simulink model "Bonus_1"  (R2024a)
settings: Solver=VariableStepAuto  StartTime=0.0  StopTime=10.0  RelTol=1e-3
libraries: HS_lib x124
settings Model: Creator=Anna  LastModifiedBy=Anna

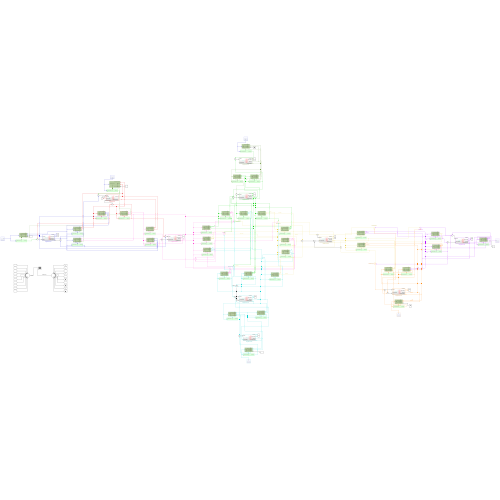
[thumbnail: Simulink's stored preview of the top-level diagram]
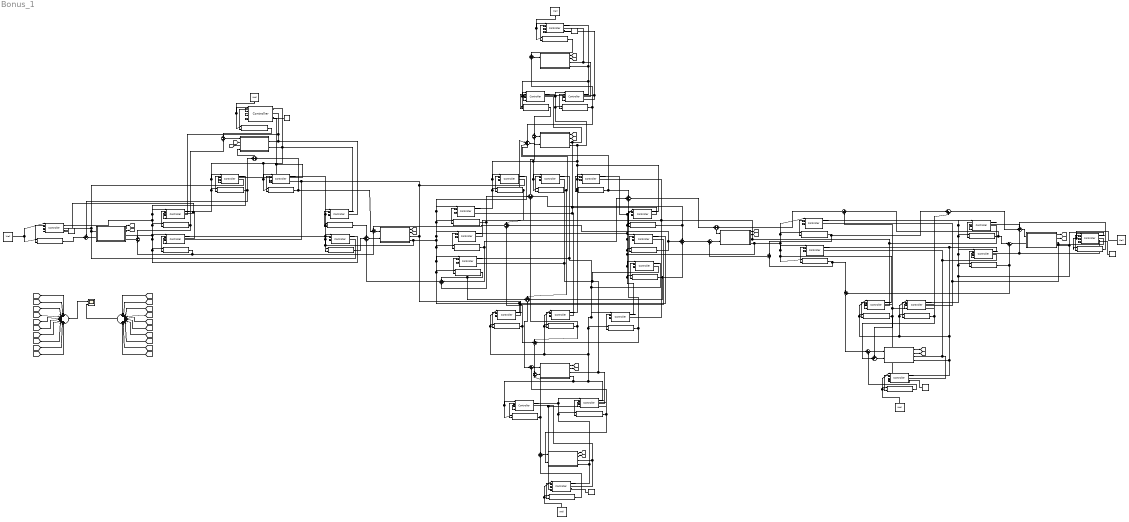
== system Bonus_1 ==
  Constant{,1..5} (6 alike) : Constant  Value=0
  Controller{1..34} (34 alike) : HS_lib/Controller  cn=0.4  cc=0.8  lb=0  ub=0
  From : From
  Goto2 : Goto
  INtakeYellow : Sum  Inputs=+++
  IntakeCyan : Sum  Inputs=+++
  IntakeGreen : Sum  Inputs=+++
  IntakeOrange : Sum  Inputs=|++
  IntakePink : Sum  Inputs=+++
  IntakeYellow2 : Sum  Inputs=|++
  Neighbourhood : Subsystem
      settings: PortSchema="{\"entries\":[{\"content\":{\"sides\":[{\"content\":{\"connectorIds\":[\"In1\",\"Out3\",\"Out4\",\"In2\"]},\"type\":\"ConnectorPlacement.EquallySpacedRectSide\",\"uuid\":\"a17f8f71-e2c0-4de1-9750-936e5df60ae2\"},{\"content\":{\"connectorIds\":[\"Out1\",\"Out2\"],\"side\":\"RIGHT\"},\"type\":\"ConnectorPlacement.EquallySpacedRectSide\",\"uuid\":\"d3f9e035-ab5e-46ba-a0b5-1d6a292e4fd8\"},{\"content\":{\"side\":\"TOP\"},\"type\":\"ConnectorPlacement.EquallySpacedRectSide\",\"uuid\":\"a414f663-cf97-4db1-b609-5e1d2eca4ce6\"}]},\"type\":\"ConnectorPlacement.EquallySpacedConnector\",\"uuid\":\"06d4f643-b53e-4a59-8698-2a41eae53feb\"}],\"packageUris\":[\"http://schema.mathworks.com/mf0/Connector/R2020b\"],\"version\":\"1.0\"}"
  Neighbourhood1 : Subsystem
      settings: PortSchema="{\"entries\":[{\"content\":{\"sides\":[{\"content\":{\"connectorIds\":[\"Out4\",\"In1\"]},\"type\":\"ConnectorPlacement.EquallySpacedRectSide\",\"uuid\":\"a17f8f71-e2c0-4de1-9750-936e5df60ae2\"},{\"content\":{\"connectorIds\":[\"Out1\",\"Out2\",\"Out3\",\"In2\"],\"side\":\"RIGHT\"},\"type\":\"ConnectorPlacement.EquallySpacedRectSide\",\"uuid\":\"d3f9e035-ab5e-46ba-a0b5-1d6a292e4fd8\"},{\"content\":{\"side\":\"TOP\"},\"type\":\"ConnectorPlacement.EquallySpacedRectSide\",\"uuid\":\"a414f663-cf97-4db1-b609-5e1d2eca4ce6\"}]},\"type\":\"ConnectorPlacement.EquallySpacedConnector\",\"uuid\":\"06d4f643-b53e-4a59-8698-2a41eae53feb\"}],\"packageUris\":[\"http://schema.mathworks.com/mf0/Connector/R2020b\"],\"version\":\"1.0\"}"
  Neighbourhood2 : Subsystem
  Neighbourhood3 : Subsystem
  Neighbourhood4 : Subsystem
  Neighbourhood5 : Subsystem
  Neighbourhood6 : Subsystem
  Neighbourhood7 : Subsystem
  Neighbourhood8 : Subsystem
  Neighbourhood9 : Subsystem
  Pump{1..34} (34 alike) : HS_lib/Pump  p=0
  Scope : Scope  NumInputPorts=2
  Sum{,1..2,7,9..10,12,14,17} (9 alike) : Sum
  Sum{11,13,16,19} (4 alike) : Sum  Inputs=|++
  Sum{4..6,15} (4 alike) : Sum  Inputs=+++
  Sum18 : Sum  Inputs=++|
  Sum20 : Sum  Inputs=++|
  Sum21 : Sum  Inputs=++++++++++
  Sum22 : Sum  Inputs=++++++++++
  Sum3 : Sum  Inputs=++|
  Sum8 : Sum  Inputs=++++
  Takeout : Sum  Inputs=+++
  Well{1..6} (6 alike) : HS_lib/Well  SystemSampleTime=-1  VariantActivationTime=update diagram  AllowFlexibleInterface=on  Latency=0  AutoFrameSizeCalculation=off
  intakeViolett : Sum  Inputs=|++
  wires:
  Controller1/1 -> Pump1/2
  Well1/1 -> Pump1/1, Controller1/1
  Neighbourhood/2(availableWater) -> Controller3/1, Pump3/1, Controller2/1, Controller6/2, Pump2/1, Controller7/2, Controller1/2  "aW"
  Neighbourhood/1(demand) -> Controller7/3, Controller6/3, Controller1/3
  Sum/1 -> Neighbourhood/2(PumpOuttake)
  Neighbourhood/3(Overflow) -> [B]
  Neighbourhood/4(notProvided) -> [b]
  Sum1/1 -> Neighbourhood/1(Intake)
  Pump1/1 -> Sum1/1
  Controller2/1 -> Pump2/2
  Controller3/1 -> Pump3/2
  Pump2/1 -> Sum/1, Sum3/1
  Pump3/1 -> Sum4/2, Sum/2
  Sum2/1 -> Neighbourhood1/2(TankFeedback)
  Pump6/1 -> Sum2/1, Sum1/2
  Controller4/1 -> Pump4/2
  Pump5/1 -> Sum2/2, Sum4/3
  Neighbourhood1/2(notProvided) -> [a]
  Neighbourhood1/4(demand) -> Controller2/3, Controller4/3, Controller8/3
  Controller6/1 -> Pump6/2
  Neighbourhood1/3(availableWater) -> Controller8/2, Pump5/1, Controller5/1, Controller2/2, Controller6/1, Controller4/2, Pump6/1
  Well2/1 -> Controller4/1, Pump4/1
  Controller5/1 -> Pump5/2
  Sum3/1 -> Neighbourhood1/1(Intake)
  Neighbourhood1/1(Overflow) -> Goto2/1
  Pump4/1 -> Sum3/2
  Neighbourhood2/1(Overflow) -> [C]
  Controller7/1 -> Pump7/2
  Controller8/1 -> Pump8/2
  Neighbourhood2/2(notProvided) -> [c]
  Sum4/1 -> Neighbourhood2/1(Intake)
  Neighbourhood2/4(availableWater) -> Controller10/1, Pump9/1, Controller14/2, Controller9/1, Controller23/1, Controller21/2, Controller17/2, Pump23/1, Pump10/1, Controller8/1, Controller5/2, Pump7/1, Controller3/2, Controller7/1, Pump8/1  "aW"
  Neighbourhood2/3(demand) -> Controller21/3, Controller17/3, Controller5/3, Controller3/3, Controller14/3  "demand"
  Sum5/1 -> Neighbourhood2/2(PumpOuttake)
  Pump7/1 -> Sum5/1
  Pump8/1 -> Sum5/2
  Sum6/1 -> Sum5/3
  Controller10/1 -> Pump10/2
  Controller9/1 -> Pump9/2
  Neighbourhood3/1(Overflow) -> [E]
  Neighbourhood3/2(notProvided) -> [e]
  Neighbourhood4/1(Overflow) -> [D]
  Neighbourhood4/2(notProvided) -> [d]
  Controller11/1 -> Pump11/2
  Well3/1 -> Pump11/1, Controller11/1
  Sum7/1 -> Neighbourhood4/1(Intake)
  Pump11/1 -> Sum7/1
  Neighbourhood4/3(demand) -> Controller13/3, Controller11/3
  Neighbourhood4/4(availableWater) -> Pump12/1, Controller12/1, Controller13/2, Controller11/2  "aW"
  Pump9/1 -> IntakeGreen/1, Sum6/3
  Pump10/1 -> Sum6/2, INtakeYellow/2
  Controller12/1 -> Pump12/2
  Controller13/1 -> Pump13/2
  Neighbourhood3/4(availableWater) -> Controller20/2, Controller18/2, Pump16/1, Controller16/1, Controller14/1, Controller9/2, Pump14/1, Controller15/1, Pump15/1, Pump13/1, Controller13/1, Controller12/2  "aW"
  Pump12/1 -> Sum9/1
  Pump13/1 -> Sum8/1, Sum7/2
  Neighbourhood3/3(demand) -> Controller12/3, Controller9/3, Controller18/3, Controller20/3  "demand"
  Controller14/1 -> Pump14/2
  Controller15/1 -> Pump15/2
  Controller16/1 -> Pump16/2
  Controller17/1 -> Pump17/2
  Controller19/1 -> Pump19/2
  Controller18/1 -> Pump18/2
  Controller20/1 -> Pump20/2
  Controller22/1 -> Pump22/2
  Controller21/1 -> Pump21/2
  Controller23/1 -> Pump23/2
  Pump23/1 -> IntakeCyan/1, Sum6/1
  Pump14/1 -> IntakePink/1, Sum8/2
  Pump15/1 -> IntakeCyan/2, Sum8/3
  Pump16/1 -> INtakeYellow/1, Sum8/4
  Sum8/1 -> Neighbourhood3/2(PumpOuttake)
  IntakePink/1 -> Sum4/1
  Sum9/1 -> Neighbourhood3/1(Intake)
  IntakeGreen/1 -> Sum9/2
  Controller24/1 -> Pump24/2
  Controller25/1 -> Pump25/2
  Controller26/1 -> Pump26/2
  Controller27/1 -> Pump27/2
  Controller29/1 -> Pump29/2
  Controller28/1 -> Pump28/2
  Controller30/1 -> Pump30/2
  Controller31/1 -> Pump31/2
  Controller32/1 -> Pump32/2
  Well4/1 -> Controller32/1, Pump32/1
  Pump32/1 -> Sum10/2
  Sum10/1 -> Neighbourhood7/1(Intake)
  Neighbourhood7/4(availableWater) -> Controller30/2, Controller31/1, Pump31/1, Controller32/2  "aW"
  Neighbourhood7/3(demand) -> Controller32/3, Controller30/3
  Pump30/1 -> Sum12/2, Sum10/1
  Neighbourhood6/4(availableWater) -> Pump30/1, Controller30/1, Controller22/2, Controller23/2, Controller15/2, Controller19/1, Pump19/1, Controller18/1, Pump18/1, Controller17/1, Pump17/1, Controller31/2  "aW"
  Sum11/1 -> Neighbourhood6/1(Intake)
  Pump31/1 -> Sum11/2, Neighbourhood7/2(PumpOuttake)
  Neighbourhood6/3(demand) -> Controller22/3, Controller23/3, Controller15/3, Controller31/3  "demand"
  Neighbourhood6/1(Overflow) -> [F]
  Neighbourhood6/2(notProvided) -> [f]
  Neighbourhood7/1(Overflow) -> [G]
  Neighbourhood7/2(notProvided) -> [g]
  IntakeCyan/1 -> Sum11/1
  Sum12/1 -> Neighbourhood6/2(PumpOuttake)
  Takeout/1 -> Sum12/1
  Pump17/1 -> Takeout/1, IntakePink/3
  Pump18/1 -> Takeout/2, IntakeGreen/2
  Pump19/1 -> Takeout/3, INtakeYellow/3
  Pump22/1 -> Sum15/3, IntakeCyan/3  "takeout3"
  Neighbourhood5/1(Overflow) -> [G2]
  Neighbourhood5/2(notProvided) -> [g2]
  Sum13/1 -> Neighbourhood5/2(PumpOuttake)
  Sum14/1 -> Sum13/2
  Sum15/1 -> Sum13/1
  Pump20/1 -> Sum15/1, IntakeGreen/3  "takeout1"
  Pump21/1 -> IntakePink/2, Sum15/2  "takeout2"
  Neighbourhood5/4(availableWater) -> Pump24/1, Controller24/1, Controller25/1, Controller26/2, Pump25/1, Controller21/1, Controller16/2, Controller20/1, Pump20/1, Controller10/2, Pump21/1, Controller19/2, Pump22/1, Controller22/1  "aW"
  Sum17/1 -> Neighbourhood5/1(Intake)
  INtakeYellow/1 -> Sum17/1
  Neighbourhood5/3(demand) -> Controller16/3, Controller10/3, Controller19/3, Controller29/3, Controller26/3  "demand"
  Pump24/1 -> intakeViolett/1, Sum14/1
  Pump25/1 -> IntakeOrange/1, Sum14/2
  Controller33/1 -> Pump33/2
  Well5/1 -> Controller33/1, Pump33/1
  Pump33/1 -> Sum19/2
  Neighbourhood8/1(Overflow) -> [H]
  Neighbourhood8/2(notProvided) -> [h]
  Neighbourhood8/3(demand) -> Controller25/3, Controller28/3, Controller33/3  "demand"
  Neighbourhood8/4(availableWater) -> Pump27/1, Controller27/1, Controller26/1, Pump26/1, Controller25/2, Controller28/2, Controller33/2  "aW"
  Controller34/1 -> Pump34/2
  Neighbourhood9/4(availableWater) -> Controller24/2, Controller29/1, Pump29/1, Controller28/1, Pump28/1, Controller27/2, Controller34/2  "aW"
  Neighbourhood9/3(demand) -> Controller34/3, Controller27/3, Controller24/3  "demand"
  Well6/1 -> Pump34/1, Controller34/1
  Pump29/1 -> IntakeYellow2/1, Sum16/1
  Sum16/1 -> Neighbourhood9/2(PumpOuttake)
  Pump28/1 -> IntakeOrange/2, Sum16/2
  Pump34/1 -> Sum18/1
  Sum18/1 -> Neighbourhood9/1(Intake)
  intakeViolett/1 -> Sum18/2
  IntakeYellow2/1 -> Sum17/2
  Sum19/1 -> Neighbourhood8/1(Intake)
  IntakeOrange/1 -> Sum19/1
  Pump26/1 -> IntakeYellow2/2, Sum20/1
  Sum20/1 -> Neighbourhood8/2(PumpOuttake)
  Pump27/1 -> Sum20/2, intakeViolett/2
  Neighbourhood9/1(Overflow) -> [I]
  Neighbourhood9/2(notProvided) -> [i]
  From/1 -> Sum21/1
  [B] -> Sum21/2
  [C] -> Sum21/3
  [D] -> Sum21/4
  [E] -> Sum21/5
  [F] -> Sum21/6
  [G2] -> Sum21/7
  [G] -> Sum21/8
  [H] -> Sum21/9
  [e] -> Sum22/5
  [f] -> Sum22/6
  [g2] -> Sum22/8
  [h] -> Sum22/9
  [a] -> Sum22/1
  [c] -> Sum22/3
  [d] -> Sum22/4
  [b] -> Sum22/2
  [g] -> Sum22/7
  [I] -> Sum21/10
  [i] -> Sum22/10
  Sum21/1 -> Scope/1  "overflow"
  Sum22/1 -> Scope/2  "notProvided"
  Constant/1 -> Controller1/4
  Constant1/1 -> Controller11/4
  Constant2/1 -> Controller34/4
  Constant3/1 -> Controller33/4
  Constant4/1 -> Controller32/4
  Constant5/1 -> Controller4/4
  Controller4/2 -> Controller5/4, Controller6/4
  Controller1/2 -> Controller3/4, Controller2/4
  Controller11/2 -> Controller12/4, Controller13/4
  Controller34/2 -> Controller29/4, Controller28/4
  Controller33/2 -> Controller26/4, Controller27/4
  Controller32/2 -> Controller31/4, Controller30/4

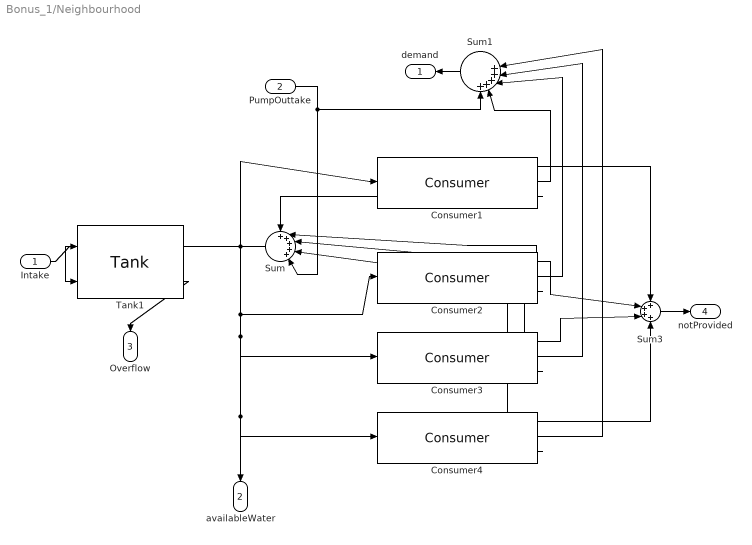
== system Bonus_1/Neighbourhood ==
  Intake : Inport
  PumpOuttake : Inport  Port=2
  Consumer{1..4} (4 alike) : HS_lib/Consumer  a=0  f=0  d=0
  Sum : Sum  Inputs=+++++|
  Sum1 : Sum  Inputs=|||+++++
  Sum3 : Sum  Inputs=++++
  Tank1 : HS_lib/Tank  c_init=0  c=100
  demand : Outport
  availableWater : Outport  Port=2
  Overflow : Outport  Port=3
  notProvided : Outport  Port=4
  wires:
  Sum/1 -> Tank1/2
  Tank1/1 -> Consumer1/1, Consumer2/1, Consumer3/1, availableWater/1, Consumer4/1
  Consumer1/2 -> Sum1/4
  Consumer2/2 -> Sum1/3
  Consumer3/2 -> Sum1/2
  Consumer4/2 -> Sum1/1
  PumpOuttake/1 -> Sum/5, Sum1/5
  Consumer2/3 -> Sum/2
  Consumer1/3 -> Sum/1
  Consumer3/3 -> Sum/3
  Consumer4/3 -> Sum/4
  Tank1/2 -> Overflow/1
  Intake/1 -> Tank1/1
  Consumer1/1 -> Sum3/1
  Consumer2/1 -> Sum3/2
  Consumer3/1 -> Sum3/3
  Consumer4/1 -> Sum3/4
  Sum3/1 -> notProvided/1
  Sum1/1 -> demand/1

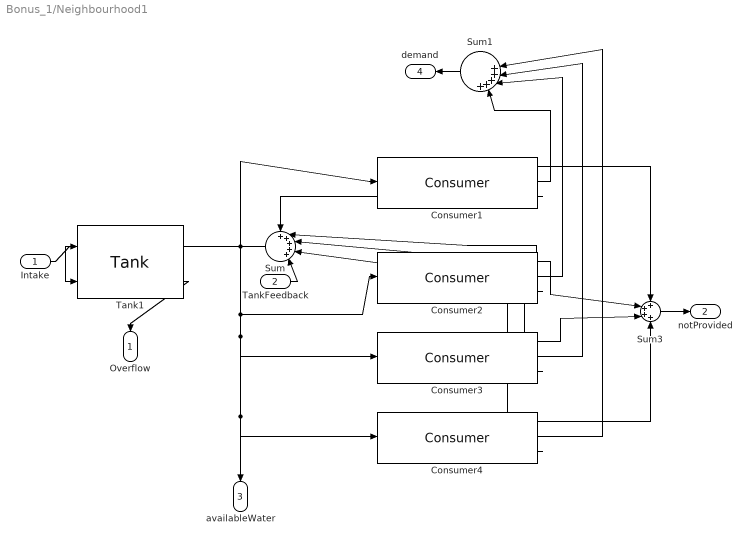
== system Bonus_1/Neighbourhood1 ==
  Intake : Inport
  TankFeedback : Inport  Port=2
  Consumer{1..4} (4 alike) : HS_lib/Consumer  a=0  f=0  d=0
  Sum : Sum  Inputs=+++++|
  Sum1 : Sum  Inputs=|||+++++
  Sum3 : Sum  Inputs=++++
  Tank1 : HS_lib/Tank  c_init=0  c=100
  Overflow : Outport
  notProvided : Outport  Port=2
  availableWater : Outport  Port=3
  demand : Outport  Port=4
  wires:
  Sum/1 -> Tank1/2
  Tank1/1 -> Consumer1/1, Consumer2/1, Consumer3/1, availableWater/1, Consumer4/1
  Consumer1/2 -> Sum1/4
  Consumer2/2 -> Sum1/3
  Consumer3/2 -> Sum1/2
  Consumer4/2 -> Sum1/1
  TankFeedback/1 -> Sum/5
  Consumer2/3 -> Sum/2
  Consumer1/3 -> Sum/1
  Consumer3/3 -> Sum/3
  Consumer4/3 -> Sum/4
  Tank1/2 -> Overflow/1
  Intake/1 -> Tank1/1
  Consumer1/1 -> Sum3/1
  Consumer2/1 -> Sum3/2
  Consumer3/1 -> Sum3/3
  Consumer4/1 -> Sum3/4
  Sum3/1 -> notProvided/1
  Sum1/1 -> demand/1

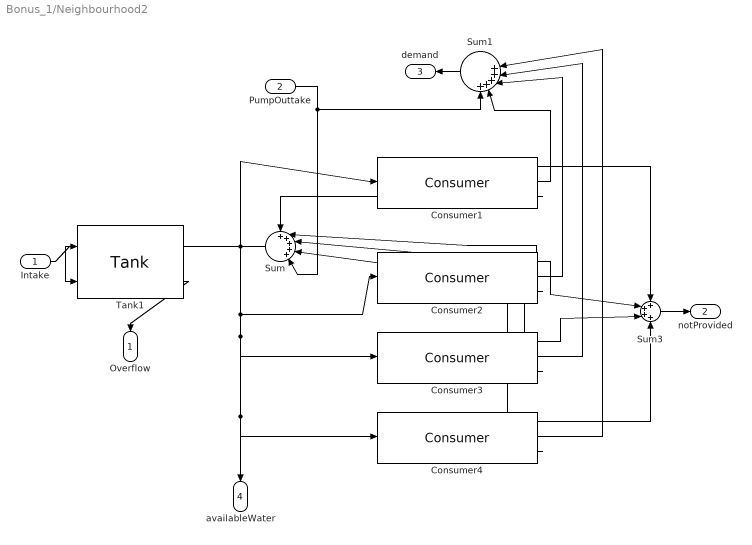
== system Bonus_1/Neighbourhood2 ==
  Intake : Inport
  PumpOuttake : Inport  Port=2
  Consumer{1..4} (4 alike) : HS_lib/Consumer  a=0  f=0  d=0
  Sum : Sum  Inputs=+++++|
  Sum1 : Sum  Inputs=|||+++++
  Sum3 : Sum  Inputs=++++
  Tank1 : HS_lib/Tank  c_init=0  c=100
  Overflow : Outport
  notProvided : Outport  Port=2
  demand : Outport  Port=3
  availableWater : Outport  Port=4
  wires:
  Sum/1 -> Tank1/2
  Tank1/1 -> Consumer1/1, Consumer2/1, Consumer3/1, availableWater/1, Consumer4/1
  Consumer1/2 -> Sum1/4
  Consumer2/2 -> Sum1/3
  Consumer3/2 -> Sum1/2
  Consumer4/2 -> Sum1/1
  PumpOuttake/1 -> Sum/5, Sum1/5
  Consumer2/3 -> Sum/2
  Consumer1/3 -> Sum/1
  Consumer3/3 -> Sum/3
  Consumer4/3 -> Sum/4
  Tank1/2 -> Overflow/1
  Intake/1 -> Tank1/1
  Consumer1/1 -> Sum3/1
  Consumer2/1 -> Sum3/2
  Consumer3/1 -> Sum3/3
  Consumer4/1 -> Sum3/4
  Sum3/1 -> notProvided/1
  Sum1/1 -> demand/1

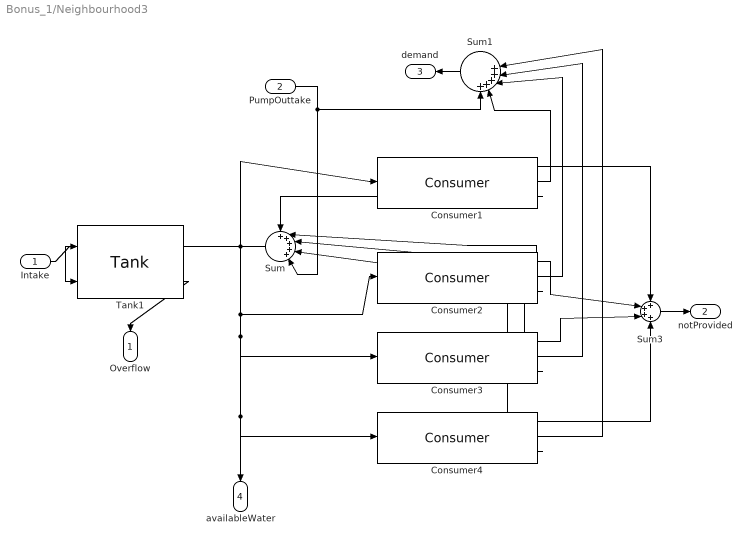
== system Bonus_1/Neighbourhood3 ==
  Intake : Inport
  PumpOuttake : Inport  Port=2
  Consumer{1..4} (4 alike) : HS_lib/Consumer  a=0  f=0  d=0
  Sum : Sum  Inputs=+++++|
  Sum1 : Sum  Inputs=|||+++++
  Sum3 : Sum  Inputs=++++
  Tank1 : HS_lib/Tank  c_init=0  c=100
  Overflow : Outport
  notProvided : Outport  Port=2
  demand : Outport  Port=3
  availableWater : Outport  Port=4
  wires:
  Sum/1 -> Tank1/2
  Tank1/1 -> Consumer1/1, Consumer2/1, Consumer3/1, availableWater/1, Consumer4/1
  Consumer1/2 -> Sum1/4
  Consumer2/2 -> Sum1/3
  Consumer3/2 -> Sum1/2
  Consumer4/2 -> Sum1/1
  PumpOuttake/1 -> Sum/5, Sum1/5
  Consumer2/3 -> Sum/2
  Consumer1/3 -> Sum/1
  Consumer3/3 -> Sum/3
  Consumer4/3 -> Sum/4
  Tank1/2 -> Overflow/1
  Intake/1 -> Tank1/1
  Consumer1/1 -> Sum3/1
  Consumer2/1 -> Sum3/2
  Consumer3/1 -> Sum3/3
  Consumer4/1 -> Sum3/4
  Sum3/1 -> notProvided/1
  Sum1/1 -> demand/1

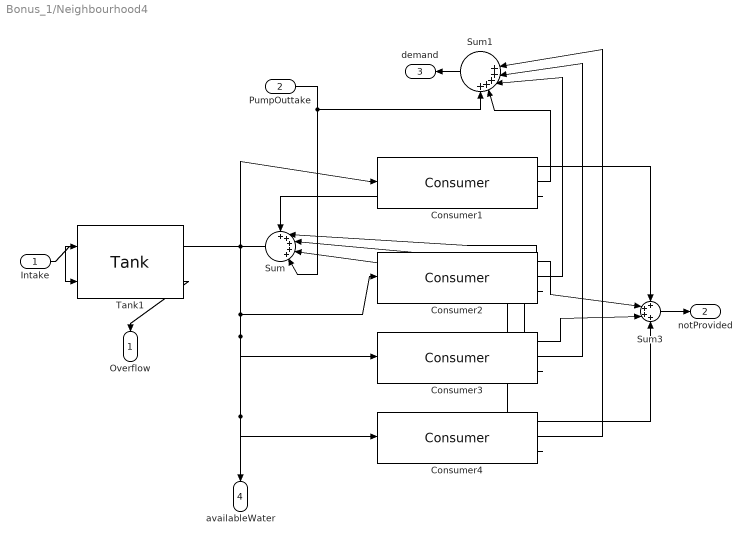
== system Bonus_1/Neighbourhood4 ==
  Intake : Inport
  PumpOuttake : Inport  Port=2
  Consumer{1..4} (4 alike) : HS_lib/Consumer  a=0  f=0  d=0
  Sum : Sum  Inputs=+++++|
  Sum1 : Sum  Inputs=|||+++++
  Sum3 : Sum  Inputs=++++
  Tank1 : HS_lib/Tank  c_init=0  c=100
  Overflow : Outport
  notProvided : Outport  Port=2
  demand : Outport  Port=3
  availableWater : Outport  Port=4
  wires:
  Sum/1 -> Tank1/2
  Tank1/1 -> Consumer1/1, Consumer2/1, Consumer3/1, availableWater/1, Consumer4/1
  Consumer1/2 -> Sum1/4
  Consumer2/2 -> Sum1/3
  Consumer3/2 -> Sum1/2
  Consumer4/2 -> Sum1/1
  PumpOuttake/1 -> Sum/5, Sum1/5
  Consumer2/3 -> Sum/2
  Consumer1/3 -> Sum/1
  Consumer3/3 -> Sum/3
  Consumer4/3 -> Sum/4
  Tank1/2 -> Overflow/1
  Intake/1 -> Tank1/1
  Consumer1/1 -> Sum3/1
  Consumer2/1 -> Sum3/2
  Consumer3/1 -> Sum3/3
  Consumer4/1 -> Sum3/4
  Sum3/1 -> notProvided/1
  Sum1/1 -> demand/1

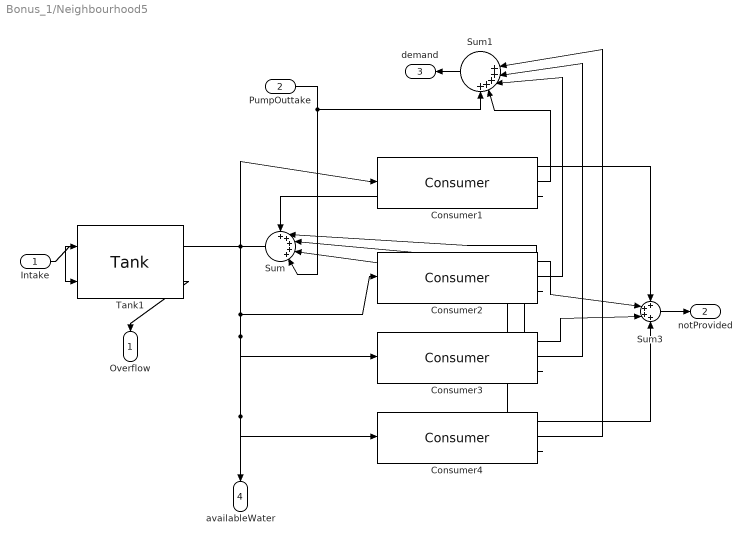
== system Bonus_1/Neighbourhood5 ==
  Intake : Inport
  PumpOuttake : Inport  Port=2
  Consumer{1..4} (4 alike) : HS_lib/Consumer  a=0  f=0  d=0
  Sum : Sum  Inputs=+++++|
  Sum1 : Sum  Inputs=|||+++++
  Sum3 : Sum  Inputs=++++
  Tank1 : HS_lib/Tank  c_init=0  c=100
  Overflow : Outport
  notProvided : Outport  Port=2
  demand : Outport  Port=3
  availableWater : Outport  Port=4
  wires:
  Sum/1 -> Tank1/2
  Tank1/1 -> Consumer1/1, Consumer2/1, Consumer3/1, availableWater/1, Consumer4/1
  Consumer1/2 -> Sum1/4
  Consumer2/2 -> Sum1/3
  Consumer3/2 -> Sum1/2
  Consumer4/2 -> Sum1/1
  PumpOuttake/1 -> Sum/5, Sum1/5
  Consumer2/3 -> Sum/2
  Consumer1/3 -> Sum/1
  Consumer3/3 -> Sum/3
  Consumer4/3 -> Sum/4
  Tank1/2 -> Overflow/1
  Intake/1 -> Tank1/1
  Consumer1/1 -> Sum3/1
  Consumer2/1 -> Sum3/2
  Consumer3/1 -> Sum3/3
  Consumer4/1 -> Sum3/4
  Sum3/1 -> notProvided/1
  Sum1/1 -> demand/1

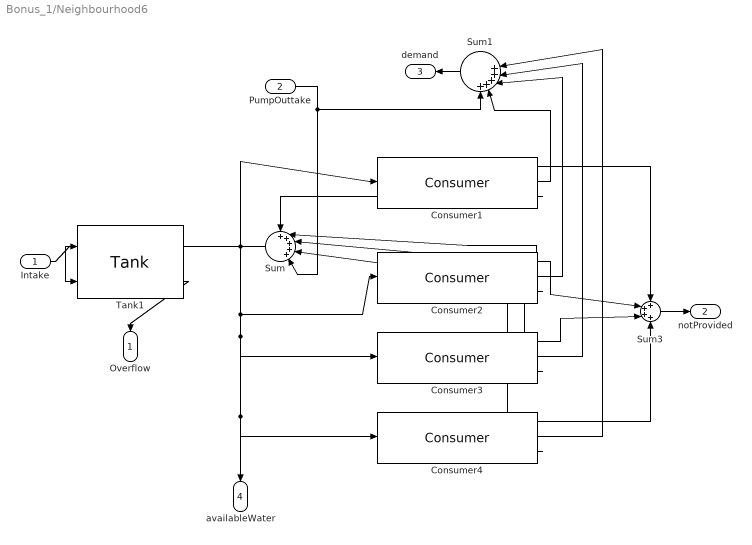
== system Bonus_1/Neighbourhood6 ==
  Intake : Inport
  PumpOuttake : Inport  Port=2
  Consumer{1..4} (4 alike) : HS_lib/Consumer  a=0  f=0  d=0
  Sum : Sum  Inputs=+++++|
  Sum1 : Sum  Inputs=|||+++++
  Sum3 : Sum  Inputs=++++
  Tank1 : HS_lib/Tank  c_init=0  c=100
  Overflow : Outport
  notProvided : Outport  Port=2
  demand : Outport  Port=3
  availableWater : Outport  Port=4
  wires:
  Sum/1 -> Tank1/2
  Tank1/1 -> Consumer1/1, Consumer2/1, Consumer3/1, availableWater/1, Consumer4/1
  Consumer1/2 -> Sum1/4
  Consumer2/2 -> Sum1/3
  Consumer3/2 -> Sum1/2
  Consumer4/2 -> Sum1/1
  PumpOuttake/1 -> Sum/5, Sum1/5
  Consumer2/3 -> Sum/2
  Consumer1/3 -> Sum/1
  Consumer3/3 -> Sum/3
  Consumer4/3 -> Sum/4
  Tank1/2 -> Overflow/1
  Intake/1 -> Tank1/1
  Consumer1/1 -> Sum3/1
  Consumer2/1 -> Sum3/2
  Consumer3/1 -> Sum3/3
  Consumer4/1 -> Sum3/4
  Sum3/1 -> notProvided/1
  Sum1/1 -> demand/1

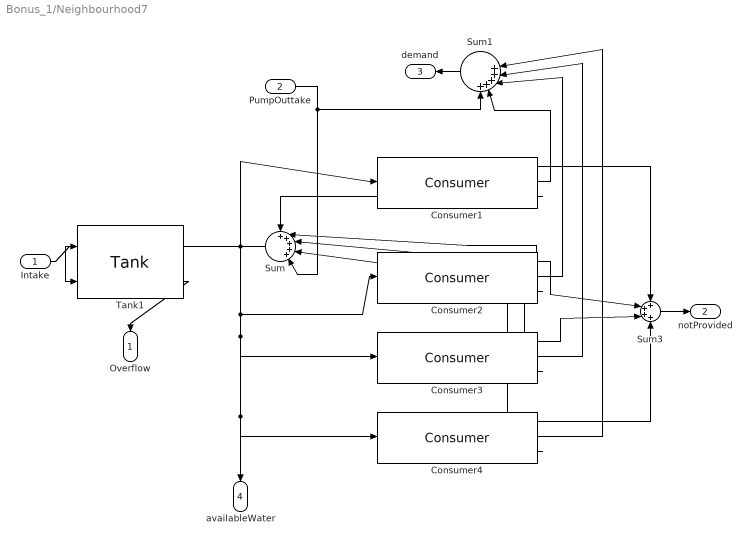
== system Bonus_1/Neighbourhood7 ==
  Intake : Inport
  PumpOuttake : Inport  Port=2
  Consumer{1..4} (4 alike) : HS_lib/Consumer  a=0  f=0  d=0
  Sum : Sum  Inputs=+++++|
  Sum1 : Sum  Inputs=|||+++++
  Sum3 : Sum  Inputs=++++
  Tank1 : HS_lib/Tank  c_init=0  c=100
  Overflow : Outport
  notProvided : Outport  Port=2
  demand : Outport  Port=3
  availableWater : Outport  Port=4
  wires:
  Sum/1 -> Tank1/2
  Tank1/1 -> Consumer1/1, Consumer2/1, Consumer3/1, availableWater/1, Consumer4/1
  Consumer1/2 -> Sum1/4
  Consumer2/2 -> Sum1/3
  Consumer3/2 -> Sum1/2
  Consumer4/2 -> Sum1/1
  PumpOuttake/1 -> Sum/5, Sum1/5
  Consumer2/3 -> Sum/2
  Consumer1/3 -> Sum/1
  Consumer3/3 -> Sum/3
  Consumer4/3 -> Sum/4
  Tank1/2 -> Overflow/1
  Intake/1 -> Tank1/1
  Consumer1/1 -> Sum3/1
  Consumer2/1 -> Sum3/2
  Consumer3/1 -> Sum3/3
  Consumer4/1 -> Sum3/4
  Sum3/1 -> notProvided/1
  Sum1/1 -> demand/1

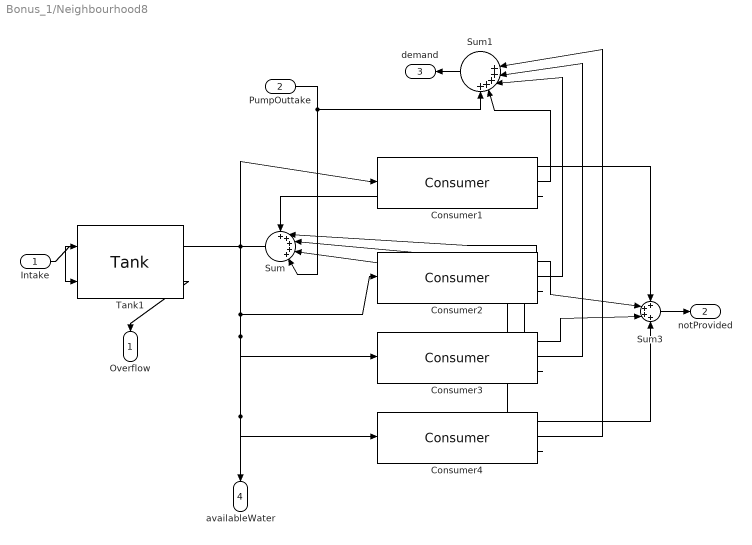
== system Bonus_1/Neighbourhood8 ==
  Intake : Inport
  PumpOuttake : Inport  Port=2
  Consumer{1..4} (4 alike) : HS_lib/Consumer  a=0  f=0  d=0
  Sum : Sum  Inputs=+++++|
  Sum1 : Sum  Inputs=|||+++++
  Sum3 : Sum  Inputs=++++
  Tank1 : HS_lib/Tank  c_init=0  c=100
  Overflow : Outport
  notProvided : Outport  Port=2
  demand : Outport  Port=3
  availableWater : Outport  Port=4
  wires:
  Sum/1 -> Tank1/2
  Tank1/1 -> Consumer1/1, Consumer2/1, Consumer3/1, availableWater/1, Consumer4/1
  Consumer1/2 -> Sum1/4
  Consumer2/2 -> Sum1/3
  Consumer3/2 -> Sum1/2
  Consumer4/2 -> Sum1/1
  PumpOuttake/1 -> Sum/5, Sum1/5
  Consumer2/3 -> Sum/2
  Consumer1/3 -> Sum/1
  Consumer3/3 -> Sum/3
  Consumer4/3 -> Sum/4
  Tank1/2 -> Overflow/1
  Intake/1 -> Tank1/1
  Consumer1/1 -> Sum3/1
  Consumer2/1 -> Sum3/2
  Consumer3/1 -> Sum3/3
  Consumer4/1 -> Sum3/4
  Sum3/1 -> notProvided/1
  Sum1/1 -> demand/1

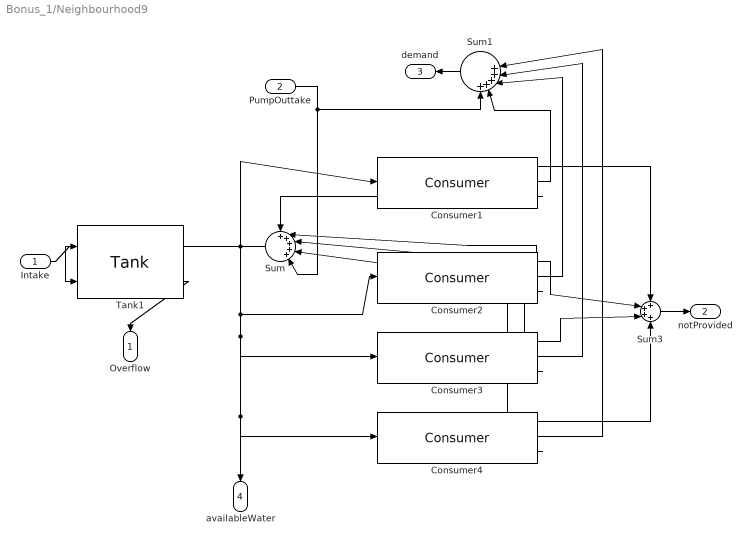
== system Bonus_1/Neighbourhood9 ==
  Intake : Inport
  PumpOuttake : Inport  Port=2
  Consumer{1..4} (4 alike) : HS_lib/Consumer  a=0  f=0  d=0
  Sum : Sum  Inputs=+++++|
  Sum1 : Sum  Inputs=|||+++++
  Sum3 : Sum  Inputs=++++
  Tank1 : HS_lib/Tank  c_init=0  c=100
  Overflow : Outport
  notProvided : Outport  Port=2
  demand : Outport  Port=3
  availableWater : Outport  Port=4
  wires:
  Sum/1 -> Tank1/2
  Tank1/1 -> Consumer1/1, Consumer2/1, Consumer3/1, availableWater/1, Consumer4/1
  Consumer1/2 -> Sum1/4
  Consumer2/2 -> Sum1/3
  Consumer3/2 -> Sum1/2
  Consumer4/2 -> Sum1/1
  PumpOuttake/1 -> Sum/5, Sum1/5
  Consumer2/3 -> Sum/2
  Consumer1/3 -> Sum/1
  Consumer3/3 -> Sum/3
  Consumer4/3 -> Sum/4
  Tank1/2 -> Overflow/1
  Intake/1 -> Tank1/1
  Consumer1/1 -> Sum3/1
  Consumer2/1 -> Sum3/2
  Consumer3/1 -> Sum3/3
  Consumer4/1 -> Sum3/4
  Sum3/1 -> notProvided/1
  Sum1/1 -> demand/1
